simulink model "IMU_INS_States"  (R2023b)
settings: Solver=VariableStepAuto  StartTime=0.0  StopTime=106  RelTol=1e-3
undefined symbols (not defined in the file or in its folder): DiscIntNeverNeededParam, fractalcoef
libraries: sim3dautolib x3, simulink x3, mspsensorlib x1, sensorinslib x1, sim3dlib x1
settings Model: SimulationMode=accelerator  PacingRate=20  Creator=Hazem Abdelaziz  LastModifiedBy=Hazem Abdelaziz

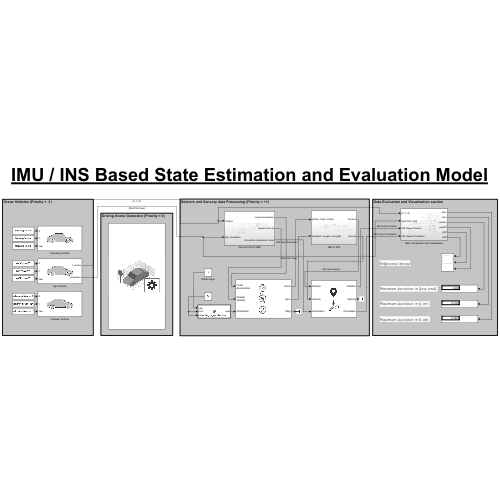
[thumbnail: Simulink's stored preview of the top-level diagram]
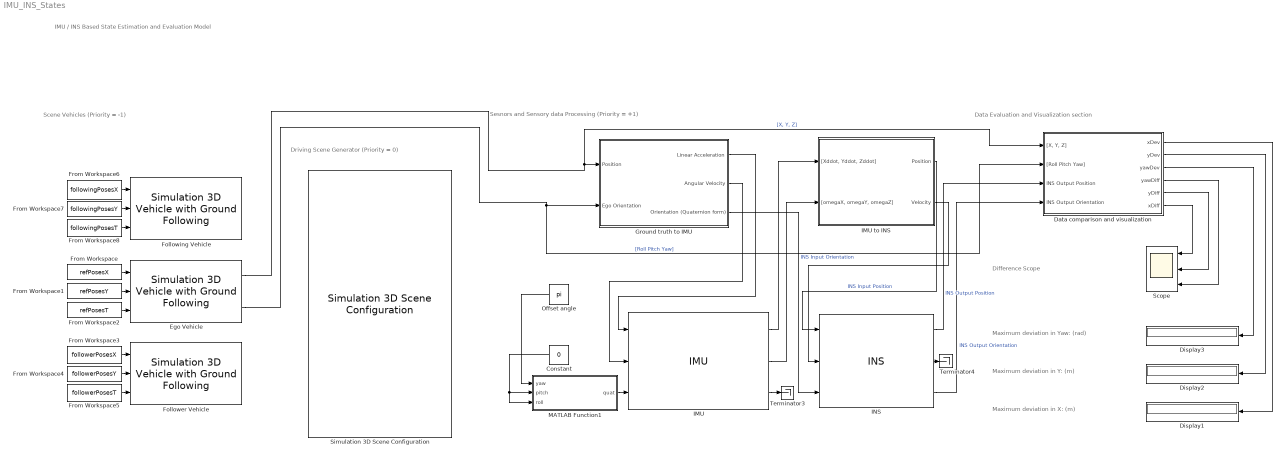
== system IMU_INS_States ==
  note: Data Evaluation and Visualization section
  note: Sesnors and Sensory data Processing (Priority = +1)
  note: Scene Vehicles (Priority = -1)
  note: Driving Scene Generator (Priority = 0)
  note: IMU / INS Based State Estimation and Evaluation Model
  note: Maximum deviation in X: (m)
  note: Maximum deviation in Y: (m)
  note: Maximum deviation in Yaw: (rad)
  note: Difference Scope
  Constant : Constant  Priority=1  Value=0
  Data comparison and visualization : Subsystem
  Display1 : Display
  Display2 : Display
  Display3 : Display
  Ego Vehicle : sim3dautolib/Simulation 3D Vehicle with Ground Following  Priority=-1  PassVehMesh=Sedan  MeshPath=/MathWorksAutomotiveContent/Vehicles/Muscle/Meshes/SK_MuscleCar.SK_MuscleCar  TrackWidth=1.9  WheelBase=3  WheelRadius=0.35  VehColor=Blue  InitialPos=[0, 0, 0]  InitialRot=[0, 0, 0]  ActorName=SimulinkVehicle1  SampleTime=-1  ActorType=SimulinkVehicle  ID=1  aMode=3  ActorTag=SimulinkVehicle1  CoordinateScheme=ISO  VehLightsControl=off  HeadlightColor=[ 1, 1, 1 ]  HighBeamIntensity=100000  LowBeamIntensity=60000  HighBeamConeAngle=70  LowBeamConeAngle=70  LeftHeadlightOrientation=[ 0, 0 ]  RightHeadlightOrientation=[ 0, 0 ]  BrakelightIntensity=500  ReverselightIntensity=500  SignallightIntensity=500  SignallightPeriod=1  SignalPulseWidth=50  TransformOutportEnabled=on
      settings: LibrarySourceBlock=drivingsim3d/Simulation 3D Vehicle with Ground Following
  Follower Vehicle : sim3dautolib/Simulation 3D Vehicle with Ground Following  Priority=-1  PassVehMesh=Small pickup truck  MeshPath=/MathWorksAutomotiveContent/Vehicles/Muscle/Meshes/SK_MuscleCar.SK_MuscleCar  TrackWidth=1.9  WheelBase=3  WheelRadius=0.35  VehColor=Black  InitialPos=[0, 0, 0]  InitialRot=[0, 0, 0]  ActorName=SimulinkVehicle2  SampleTime=-1  ActorType=SimulinkVehicle  ID=2  aMode=3  ActorTag=SimulinkVehicle2  CoordinateScheme=ISO  VehLightsControl=off  HeadlightColor=[ 1, 1, 1 ]  HighBeamIntensity=100000  LowBeamIntensity=60000  HighBeamConeAngle=70  LowBeamConeAngle=70  LeftHeadlightOrientation=[ 0, 0 ]  RightHeadlightOrientation=[ 0, 0 ]  BrakelightIntensity=500  ReverselightIntensity=500  SignallightIntensity=500  SignallightPeriod=1  SignalPulseWidth=50  TransformOutportEnabled=off
      settings: LibrarySourceBlock=drivingsim3d/Simulation 3D Vehicle with Ground Following
  Following Vehicle : sim3dautolib/Simulation 3D Vehicle with Ground Following  Priority=-1  PassVehMesh=Box truck  MeshPath=/MathWorksAutomotiveContent/Vehicles/Muscle/Meshes/SK_MuscleCar.SK_MuscleCar  TrackWidth=1.9  WheelBase=3  WheelRadius=0.35  VehColor=White  InitialPos=[0, 0, 0]  InitialRot=[0, 0, 0]  ActorName=SimulinkVehicle3  SampleTime=-1  ActorType=SimulinkVehicle  ID=3  aMode=3  ActorTag=SimulinkVehicle3  CoordinateScheme=ISO  VehLightsControl=off  HeadlightColor=[ 1, 1, 1 ]  HighBeamIntensity=100000  LowBeamIntensity=60000  HighBeamConeAngle=70  LowBeamConeAngle=70  LeftHeadlightOrientation=[ 0, 0 ]  RightHeadlightOrientation=[ 0, 0 ]  BrakelightIntensity=500  ReverselightIntensity=500  SignallightIntensity=500  SignallightPeriod=1  SignalPulseWidth=50  TransformOutportEnabled=off
      settings: LibrarySourceBlock=drivingsim3d/Simulation 3D Vehicle with Ground Following
  From Workspace : FromWorkspace  VariableName=refPosesX
  From Workspace1 : FromWorkspace  VariableName=refPosesY
  From Workspace2 : FromWorkspace  VariableName=refPosesT
  From Workspace3 : FromWorkspace  VariableName=followerPosesX
  From Workspace4 : FromWorkspace  VariableName=followerPosesY
  From Workspace5 : FromWorkspace  VariableName=followerPosesT
  From Workspace6 : FromWorkspace  VariableName=followingPosesX
  From Workspace7 : FromWorkspace  VariableName=followingPosesY
  From Workspace8 : FromWorkspace  VariableName=followingPosesT
  Ground truth to IMU : Subsystem  Priority=1
  IMU : mspsensorlib/IMU  Priority=1  DispRefFrame=ENU  TemperaturePort=off  Temperature=25  MagneticFieldPort=off  MagneticFieldNED=[ 27.5550, -2.4169, -16.0849 ]  MagneticFieldENU=[-2.4169, 27.5550, 16.0849]  SeedDouble=0  SimulateUsing=Interpreted execution  AccelParamsMeasurementRange=Inf  AccelParamsResolution=0  AccelParamsConstantBias=[ 0, 0, 9.80 ]  AccelParamsAxesMisalignment=[ 100, 0, 0; 0, 100, 0; 0, 0, 100 ]  AccelParamsNoiseDensity=[ 0, 0, 0 ]  AccelParamsBiasInstability=[ 0, 0, 0 ]  AccelParamsBiasInstabilityNumerator=fractalcoef().Numerator  AccelParamsBiasInstabilityDenominator=fractalcoef().Denominator  AccelParamsRandomWalk=[ 0, 0, 0 ]  AccelParamsNoiseType=double-sided  AccelParamsTemperatureBias=[ 0, 0, 0 ]  AccelParamsTemperatureScaleFactor=[ 0, 0, 0 ]  GyroParamsMeasurementRange=Inf  GyroParamsResolution=0  GyroParamsConstantBias=[ 0, 0, 0 ]  GyroParamsAxesMisalignment=[ 100, 0, 0; 0, 100, 0; 0, 0, 100 ]  GyroParamsAccelerationBias=[ 0, 0, 0 ]  GyroParamsNoiseDensity=[ 0, 0, 0 ]  GyroParamsBiasInstability=[ 0, 0, 0 ]  GyroParamsBiasInstabilityNumerator=fractalcoef().Numerator  GyroParamsBiasInstabilityDenominator=fractalcoef().Denominator  GyroParamsRandomWalk=[ 0, 0, 0 ]  GyroParamsNoiseType=double-sided  GyroParamsTemperatureBias=[ 0, 0, 0 ]  GyroParamsTemperatureScaleFactor=[ 0, 0, 0 ]  MagParamsMeasurementRange=Inf  MagParamsResolution=0  MagParamsConstantBias=[ 0, 0, 0 ]  MagParamsAxesMisalignment=[ 100, 0, 0; 0, 100, 0; 0, 0, 100 ]  MagParamsNoiseDensity=[ 0, 0, 0 ]  MagParamsBiasInstability=[ 0, 0, 0 ]  MagParamsBiasInstabilityNumerator=fractalcoef().Numerator  MagParamsBiasInstabilityDenominator=fractalcoef().Denominator  MagParamsRandomWalk=[ 0, 0, 0 ]  MagParamsNoiseType=double-sided  MagParamsTemperatureBias=[ 0, 0, 0 ]  MagParamsTemperatureScaleFactor=[ 0, 0, 0 ]
  IMU to INS : Subsystem  Priority=1
  INS : sensorinslib/INS  Priority=1  MountingLocation=[0 0 0]  RollAccuracy=0.05  PitchAccuracy=0.05  YawAccuracy=0.05  PositionAccuracy=0.1  VelocityAccuracy=0.1  UseAccelAndAngVel=off  AccelerationAccuracy=0.1  AngularVelocityAccuracy=0.1  TimeInput=off  PositionErrorFactor=[0 0 0]  SeedDouble=67  SimulateUsing=Code generation
      settings: LibrarySourceBlock=mspsensorlib/INS
  MATLAB Function1 : MATLAB Function  Priority=1  TreatAsAtomicUnit=on
  Offset angle : Constant  Priority=1  Value=pi
  Scope : Scope  NumInputPorts=3
  Simulation 3D Scene Configuration : sim3dlib/Simulation 3D Scene Configuration  Priority=0  ProjectFormat=Default Scenes  SceneDesc=US city block  ProjectName=C:\Program Files\MATLAB\R2023b\toolbox\shared\sim3d_projects\automotive_project_windows\UE\WindowsNoEditor\VehicleSimulation.exe  ScenePath=/Game/Maps/HwStrght  EnableOpenDRIVE=off  vehTagList={'Custom';'Scene Origin';'SimulinkVehicle1';'SimulinkVehicle2';'SimulinkVehicle3'}  vehTag=SimulinkVehicle2  FreeCameraInitialTranslation=[0, 0, 0]  FreeCameraDefaultInitialTranslation=[-6, 0, 2]  FreeCameraInitialRotation=[0, 0, 0]  FreeCameraDefaultInitialRotation=[0, -15, 0]  OpVisEn=off  Ts=0.01  EnableWindow=on  EnableRemoteAccess=off  EnableWeather=off  SunAltitude=40.0  SunAzimuth=90  clouds=10  wind=1  fog=0  rain=0  EnableGeospatial=off  OriginHeight=200  OriginLatitude=40.744652  OriginLongitude=-73.988864  MapStyle=Aerial  AdditionalAssetIDs=[]  UseAdvancedSunSky=off  SolarTime=11  TimeZone=-5  Day=21  Month=9  Year=2022  UseDaylightSavingTime=on  DSTStartDay=10  DSTStartMonth=3  DSTEndDay=3  DSTEndMonth=11  DSTSwitchHour=2  sensorTag=MainCamera1  sensorId=1  sensorName=MainCamera1  mountLoc=Origin  offsetFlag=off  tmountOffset=[0, 0, 0]  rmountOffset=[0, 0, 0]  HorizontalResolution=1280  VerticalResolution=720  HorizontalFOV=60  mountPoint=[0 0 0]  mountOrientation=[0 0 0]  aMode=3  ID=1  GeoTrigger=Inactive
      settings: LibrarySourceBlock=drivingsim3d/Simulation 3D Scene Configuration
  Terminator3 : Terminator
  Terminator4 : Terminator
  wires:
  From Workspace/1 -> Ego Vehicle/1
  From Workspace1/1 -> Ego Vehicle/2
  From Workspace2/1 -> Ego Vehicle/3
  From Workspace3/1 -> Follower Vehicle/1
  From Workspace4/1 -> Follower Vehicle/2
  From Workspace5/1 -> Follower Vehicle/3
  From Workspace7/1 -> Following Vehicle/2
  From Workspace8/1 -> Following Vehicle/3
  From Workspace6/1 -> Following Vehicle/1
  Ground truth to IMU/2(Angular Velocity) -> IMU/2
  IMU to INS/2(Velocity) -> INS/2
  IMU to INS/1(Position) -> INS/1  "INS Input Position"
  IMU/3 -> Terminator3/1
  IMU/1 -> IMU to INS/1("[Xddot, Yddot, Zddot]")
  Ground truth to IMU/1(Linear Acceleration) -> IMU/1
  IMU/2 -> IMU to INS/2("[omegaX, omegaY, omegaZ]")
  Ego Vehicle/1 -> Data comparison and visualization/1("[X, Y, Z]"), Ground truth to IMU/1(Position)  "[X, Y, Z]"
  Ego Vehicle/2 -> Data comparison and visualization/2("[Roll Pitch Yaw]"), Ground truth to IMU/2(Ego Orientation)  "[Roll Pitch Yaw]"
  INS/2 -> Terminator4/1
  MATLAB Function1/1(quat) -> IMU/3
  Constant/1 -> MATLAB Function1/2(pitch), MATLAB Function1/3(roll)
  Ground truth to IMU/3(Orientation (Quaternion form)) -> INS/3  "INS Input Orientation"
  INS/1 -> Data comparison and visualization/3(INS Output Position)  "INS Output Position"
  INS/3 -> Data comparison and visualization/4(INS Output Orientation)  "INS Output Orientation"
  Data comparison and visualization/6(xDiff) -> Scope/1
  Data comparison and visualization/5(yDiff) -> Scope/2
  Data comparison and visualization/1(xDev) -> Display1/1
  Data comparison and visualization/2(yDev) -> Display2/1
  Data comparison and visualization/3(yawDev) -> Display3/1
  Data comparison and visualization/4(yawDiff) -> Scope/3
  Offset angle/1 -> MATLAB Function1/1(yaw)

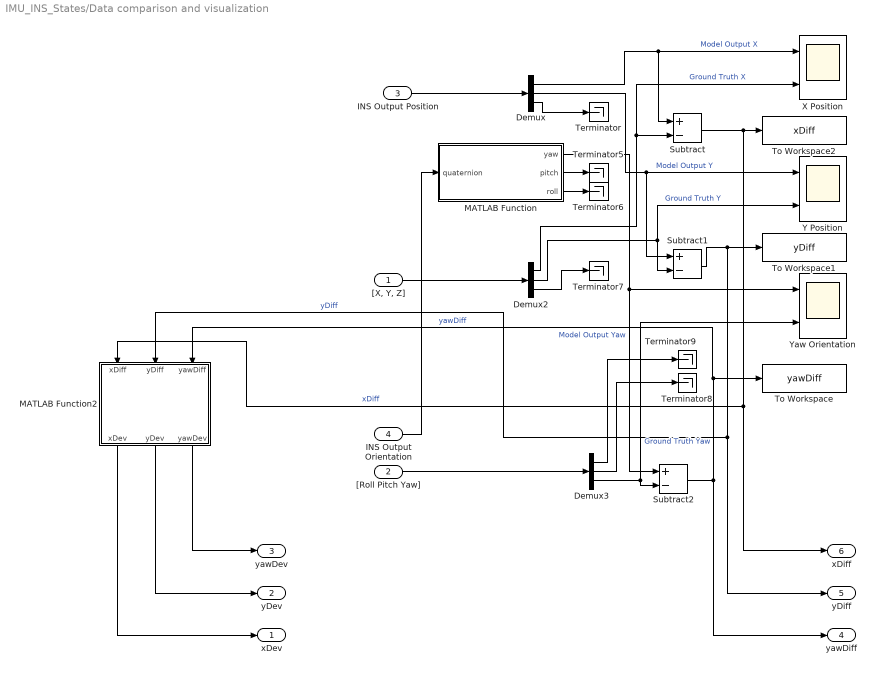
== system IMU_INS_States/Data comparison and visualization ==
  "[X, Y, Z]" : Inport
  "[Roll Pitch Yaw]" : Inport  Port=2
  INS Output Position : Inport  Port=3
  INS Output Orientation : Inport  Port=4
  Demux : Demux  Outputs=3
  Demux2 : Demux  Outputs=3
  Demux3 : Demux  Outputs=3
  MATLAB Function : MATLAB Function  TreatAsAtomicUnit=on
  MATLAB Function2 : MATLAB Function  TreatAsAtomicUnit=on
  Subtract : Sum  Inputs=+-
  Subtract1 : Sum  Inputs=+-
  Subtract2 : Sum  Inputs=+-
  Terminator{,5..9} (6 alike) : Terminator
  To Workspace : ToWorkspace  VariableName=yawDiff  SaveFormat=Timeseries  SampleTime=-1
  To Workspace1 : ToWorkspace  VariableName=yDiff  SaveFormat=Timeseries  SampleTime=-1
  To Workspace2 : ToWorkspace  VariableName=xDiff  SaveFormat=Timeseries  SampleTime=-1
  X Position : Scope  NumInputPorts=2
  Y Position : Scope  NumInputPorts=2
  Yaw Orientation : Scope  NumInputPorts=2
  xDev : Outport
  yDev : Outport  Port=2
  yawDev : Outport  Port=3
  yawDiff : Outport  Port=4
  yDiff : Outport  Port=5
  xDiff : Outport  Port=6
  wires:
  MATLAB Function/1(yaw) -> Subtract2/1, Yaw Orientation/1  "Model Output Yaw"
  Demux3/2 -> Terminator8/1
  Demux3/3 -> Subtract2/2, Yaw Orientation/2  "Ground Truth Yaw"
  Demux/1 -> X Position/1, Subtract/1  "Model Output X"
  Demux2/1 -> X Position/2, Subtract/2  "Ground Truth X"
  Subtract1/1 -> yDiff/1, MATLAB Function2/2(yDiff), To Workspace1/1  "yDiff"
  INS Output Orientation/1 -> MATLAB Function/1(quaternion)
  MATLAB Function/2(pitch) -> Terminator5/1
  Subtract/1 -> xDiff/1, MATLAB Function2/1(xDiff), To Workspace2/1  "xDiff"
  Demux/2 -> Subtract1/1, Y Position/1  "Model Output Y"
  Demux2/2 -> Subtract1/2, Y Position/2  "Ground Truth Y"
  MATLAB Function/3(roll) -> Terminator6/1
  Subtract2/1 -> yawDiff/1, MATLAB Function2/3(yawDiff), To Workspace/1  "yawDiff"
  MATLAB Function2/1(xDev) -> xDev/1
  Demux2/3 -> Terminator7/1
  INS Output Position/1 -> Demux/1
  Demux/3 -> Terminator/1
  Demux3/1 -> Terminator9/1
  "[X, Y, Z]"/1 -> Demux2/1
  "[Roll Pitch Yaw]"/1 -> Demux3/1
  MATLAB Function2/2(yDev) -> yDev/1
  MATLAB Function2/3(yawDev) -> yawDev/1

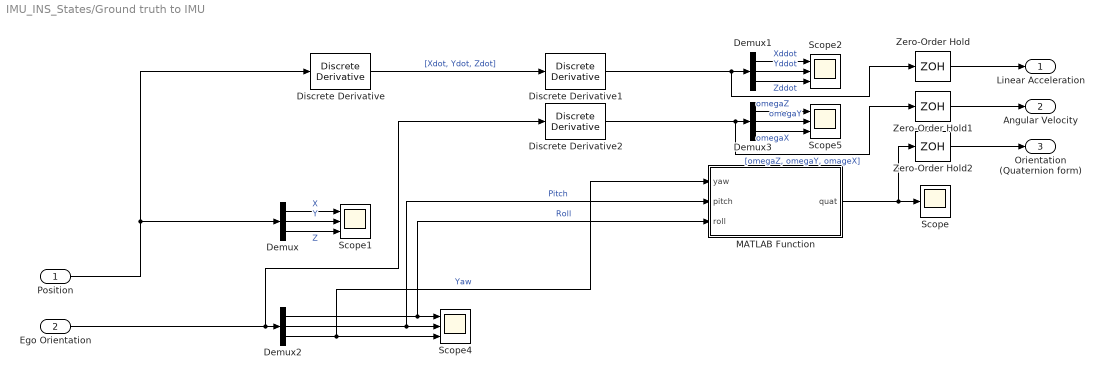
== system IMU_INS_States/Ground truth to IMU ==
  Position : Inport
  Ego Orientation : Inport  Port=2
  Demux{,1..3} (4 alike) : Demux  Outputs=3
  Discrete Derivative : simulink/Discrete/Discrete Derivative  gainval=1.0  ICPrevScaledInput=0  OutMin=[]  OutMax=[]  OutDataType=fixdt(1, 16)  OutScaling=2^-10  DoSatur=off
  Discrete Derivative1 : simulink/Discrete/Discrete Derivative  gainval=1.0  ICPrevScaledInput=0  OutMin=[]  OutMax=[]  OutDataType=fixdt(1, 16)  OutScaling=2^-10  DoSatur=off
  Discrete Derivative2 : simulink/Discrete/Discrete Derivative  gainval=1  ICPrevScaledInput=0  OutMin=[]  OutMax=[]  OutDataType=fixdt(1, 16)  OutScaling=2^-10  DoSatur=off
  MATLAB Function : MATLAB Function  TreatAsAtomicUnit=on
  Scope : Scope
  Scope{1..2,4..5} (4 alike) : Scope  NumInputPorts=3
  Zero-Order Hold : ZeroOrderHold  SampleTime=-1
  Zero-Order Hold1 : ZeroOrderHold  SampleTime=-1
  Zero-Order Hold2 : ZeroOrderHold  SampleTime=-1
  Linear Acceleration : Outport
  Angular Velocity : Outport  Port=2
  Orientation (Quaternion form) : Outport  Port=3
  wires:
  Demux1/1 -> Scope2/1  "Xddot"
  Discrete Derivative/1 -> Discrete Derivative1/1  "[Xdot, Ydot, Zdot]"
  Zero-Order Hold2/1 -> Orientation (Quaternion form)/1
  Demux2/1 -> MATLAB Function/3(roll), Scope4/1  "Roll"
  Discrete Derivative2/1 -> Zero-Order Hold1/1, Demux3/1  "[omegaZ, omegaY, omageX]"
  Ego Orientation/1 -> Discrete Derivative2/1, Demux2/1
  Demux2/3 -> MATLAB Function/1(yaw), Scope4/3  "Yaw"
  Demux1/3 -> Scope2/3  "Zddot"
  Demux2/2 -> MATLAB Function/2(pitch), Scope4/2  "Pitch"
  Discrete Derivative1/1 -> Zero-Order Hold/1, Demux1/1
  Demux3/3 -> Scope5/3  "omegaX"
  Demux/2 -> Scope1/2  "Y"
  Zero-Order Hold/1 -> Linear Acceleration/1
  Demux3/1 -> Scope5/1  "omegaZ"
  MATLAB Function/1(quat) -> Zero-Order Hold2/1, Scope/1
  Demux/1 -> Scope1/1  "X"
  Demux1/2 -> Scope2/2  "Yddot"
  Position/1 -> Discrete Derivative/1, Demux/1
  Demux3/2 -> Scope5/2  "omegaY"
  Demux/3 -> Scope1/3  "Z"
  Zero-Order Hold1/1 -> Angular Velocity/1

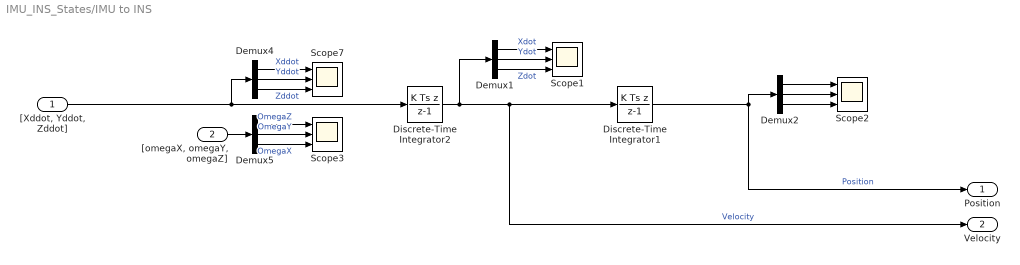
== system IMU_INS_States/IMU to INS ==
  "[Xddot, Yddot, Zddot]" : Inport
  "[omegaX, omegaY, omegaZ]" : Inport  Port=2
  Demux{1..2,4..5} (4 alike) : Demux  Outputs=3
  Discrete-Time Integrator1 : DiscreteIntegrator  Priority=-1  IntegratorMethod=Integration: Backward Euler  SampleTime=-1  RndMeth=Round  ICPrevOutput=DiscIntNeverNeededParam  ICPrevScaledInput=DiscIntNeverNeededParam
  Discrete-Time Integrator2 : DiscreteIntegrator  Priority=-1  IntegratorMethod=Integration: Backward Euler  SampleTime=-1  ICPrevOutput=DiscIntNeverNeededParam  ICPrevScaledInput=DiscIntNeverNeededParam
  Scope{1..3,7} (4 alike) : Scope  NumInputPorts=3
  Position : Outport
  Velocity : Outport  Port=2
  wires:
  Demux5/1 -> Scope3/1  "OmegaZ"
  Demux4/2 -> Scope7/2  "Yddot"
  Discrete-Time Integrator2/1 -> Velocity/1, Discrete-Time Integrator1/1, Demux1/1  "Velocity"
  Demux2/3 -> Scope2/3
  Demux4/3 -> Scope7/3  "Zddot"
  Demux5/3 -> Scope3/3  "OmegaX"
  Demux4/1 -> Scope7/1  "Xddot"
  Demux5/2 -> Scope3/2  "OmegaY"
  "[Xddot, Yddot, Zddot]"/1 -> Discrete-Time Integrator2/1, Demux4/1
  Demux2/1 -> Scope2/1
  Demux2/2 -> Scope2/2
  "[omegaX, omegaY, omegaZ]"/1 -> Demux5/1
  Demux1/3 -> Scope1/3  "Zdot"
  Demux1/1 -> Scope1/1  "Xdot"
  Demux1/2 -> Scope1/2  "Ydot"
  Discrete-Time Integrator1/1 -> Position/1, Demux2/1  "Position"

== matlab function IMU_INS_States/Ground truth to IMU/MATLAB Function ==
  data: yaw input; quat output; pitch input; roll input
function quat = euler_to_quaternion(yaw, pitch, roll)
    %Converting Euler angles to quaternion


    % Compute quaternion components
    cy = cos(yaw * 0.5);
    sy = sin(yaw * 0.5);
    cp = cos(pitch * 0.5);
    sp = sin(pitch * 0.5);
    cr = cos(roll * 0.5);
    sr = sin(roll * 0.5);

    % Quaternion elements
    qw = cy * cp * cr + sy * sp * sr;
    qx = cy * cp * sr - sy * sp * cr;
    qy = sy * cp * sr + cy * sp * cr;
    qz = sy * cp * cr - cy * sp * sr;

    % Output quaternion
    quat = [qw, qx, qy, qz];

== matlab function IMU_INS_States/Data comparison and visualization/MATLAB Function ==
  data: quaternion input; yaw output; pitch output; roll output
function [yaw, pitch ,roll] = quaternion_to_euler(quaternion)
%Converting quaternion vector to euler angles


    %Extract quaternion components
    q0 = quaternion(1);
    q1 = quaternion(2);
    q2 = quaternion(3);
    q3 = quaternion(4);

    %Euler angles
    yaw = (atan2(2*(q0*q3 + q1*q2), 1 - 2*(q2^2 + q3^2)));
    
    %for the evaluation model and to obtain continous form of yaw angle
    %that means if yaw is getting just over -pi
    % don't wrap it up to pi (as range [-pi pi]
    %instead do angle = (-pi -small_angle)
    if (yaw > pi)
        yaw = pi + mod(yaw, pi);
    elseif (yaw < -pi)
        yaw = -pi + mod(yaw, -pi);
    end
    pitch = asin(2*(q0*q2 - q3*q1));
    roll = atan2(2*(q0*q1 + q2*q3), 1 - 2*(q1^2 + q2^2));

== matlab function IMU_INS_States/MATLAB Function1 ==
  data: yaw input; quat output; pitch input; roll input
function quat = euler_to_quaternion(yaw, pitch, roll)
    %Converting Euler angles to quaternion


    % Compute quaternion components
    cy = cos(yaw * 0.5);
    sy = sin(yaw * 0.5);
    cp = cos(pitch * 0.5);
    sp = sin(pitch * 0.5);
    cr = cos(roll * 0.5);
    sr = sin(roll * 0.5);

    % Quaternion elements
    qw = cy * cp * cr + sy * sp * sr;
    qx = cy * cp * sr - sy * sp * cr;
    qy = sy * cp * sr + cy * sp * cr;
    qz = sy * cp * cr - cy * sp * sr;

    % Output quaternion
    quat = [qw, qx, qy, qz];

== matlab function IMU_INS_States/Data comparison and visualization/MATLAB Function2 ==
  data: xDiff input; xDev output; yDev output; yawDev output; yDiff input; yawDiff input
function [xDev, yDev ,yawDev] = modelEval(xDiff, yDiff, yawDiff)

    persistent x; % Declare persistent variable
    persistent y; % Declare persistent variable
    persistent yaw; % Declare persistent variable
    
    if isempty(x)
        % Initialize the persistent variable if it's empty
        x = 0;
        y = 0;
        yaw = 0;
    end

   if(abs(xDiff) > abs(x))
       x=xDiff;
   end
   if(abs(yDiff) > abs(y))
       y=yDiff;
   end
   if(abs(yawDiff) > abs(yaw))
       yaw=yawDiff;
   end
    xDev = abs(x);
    yDev = abs(y);
    yawDev = abs(yaw);
